simulink model "maquina_inducao_regime_permanente"  (R2015a)
settings: Solver=ode45  StartTime=0.0  StopTime=1.0  FixedStep=50e-6  MaxStep=50e-6  RelTol=1e-3
values from neighbouring files (symbols this model uses):
  FLrd_0 = FLr_dq_0    [MI_controle_W_I_T_inicio.m]    (also in MI_controle_W_I_inicio.m; MI_controle_W_I_startup_inicio.m; MI_controle_W_Inicio.m; MI_controle_W_T_I_startup_inicio.m)
  FLrq_0 = FluxLinkage_dq(4)    [MI_controle_W_I_T_inicio.m]    (also in MI_controle_W_I_inicio.m; MI_controle_W_I_startup_inicio.m; MI_controle_W_Inicio.m = 0; MI_controle_W_T_I_startup_inicio.m)
  FLsd_0 = FluxLinkage_dq(1)    [MI_controle_W_I_T_inicio.m]    (also in MI_controle_W_I_inicio.m; MI_controle_W_I_startup_inicio.m; MI_controle_W_Inicio.m; MI_controle_W_T_I_startup_inicio.m)
  FLsq_0 = FluxLinkage_dq(2)    [MI_controle_W_I_T_inicio.m]    (also in MI_controle_W_I_inicio.m; MI_controle_W_I_startup_inicio.m; MI_controle_W_Inicio.m; MI_controle_W_T_I_startup_inicio.m)
  J = 0.025    [MI_controle_W_I_T_inicio.m]    (also in MI_controle_W_I_inicio.m; MI_controle_W_I_startup_inicio.m; MI_controle_W_Inicio.m; MI_controle_W_T_I_startup_inicio.m)
  Lm = Xm/Wsyn    (= 0.368708951496)    [MI_controle_W_I_T_inicio.m]    (also in MI_controle_W_I_inicio.m; MI_controle_W_I_startup_inicio.m; MI_controle_W_Inicio.m; MI_controle_W_T_I_startup_inicio.m)
  Minv = inv(M)    [MI_controle_W_I_T_inicio.m]    (also in MI_controle_W_I_inicio.m; MI_controle_W_I_startup_inicio.m; MI_controle_W_Inicio.m; MI_controle_W_T_I_startup_inicio.m)
  p = 4    [MI_controle_W_I_T_inicio.m]    (also in MI_controle_W_I_inicio.m; MI_controle_W_I_startup_inicio.m; MI_controle_W_Inicio.m; MI_controle_W_T_I_startup_inicio.m)
  Rr = 1.34    [MI_controle_W_I_T_inicio.m]    (also in MI_controle_W_I_inicio.m; MI_controle_W_I_startup_inicio.m; MI_controle_W_Inicio.m; MI_controle_W_T_I_startup_inicio.m)
  Rs = 1.77    [MI_controle_W_I_T_inicio.m]    (also in MI_controle_W_I_inicio.m; MI_controle_W_I_startup_inicio.m; MI_controle_W_Inicio.m; MI_controle_W_T_I_startup_inicio.m)
  TL_0 = Tem_0    [MI_controle_W_I_T_inicio.m]    (also in MI_controle_W_I_inicio.m; MI_controle_W_I_startup_inicio.m = 0; MI_controle_W_Inicio.m; MI_controle_W_T_I_startup_inicio.m = 0)
  Va = VLLrms*sqrt(2/3)    [MI_controle_W_I_T_inicio.m]    (also in MI_controle_W_I_inicio.m; MI_controle_W_I_startup_inicio.m; MI_controle_W_Inicio.m; MI_controle_W_T_I_startup_inicio.m)
  Wmech_0 = (2/p)*(1-s)*Wsyn    (= 185.253435597)    [MI_controle_W_I_T_inicio.m]    (also in MI_controle_W_I_inicio.m; MI_controle_W_I_startup_inicio.m = 0; MI_controle_W_Inicio.m; MI_controle_W_T_I_startup_inicio.m = 0)
  Wsyn = 2*pi*f    (= 376.991118431)    [MI_controle_W_I_T_inicio.m]    (also in MI_controle_W_I_inicio.m; MI_controle_W_I_startup_inicio.m; MI_controle_W_Inicio.m; MI_controle_W_T_I_startup_inicio.m)
settings Model: Creator=range  LastModifiedBy=range

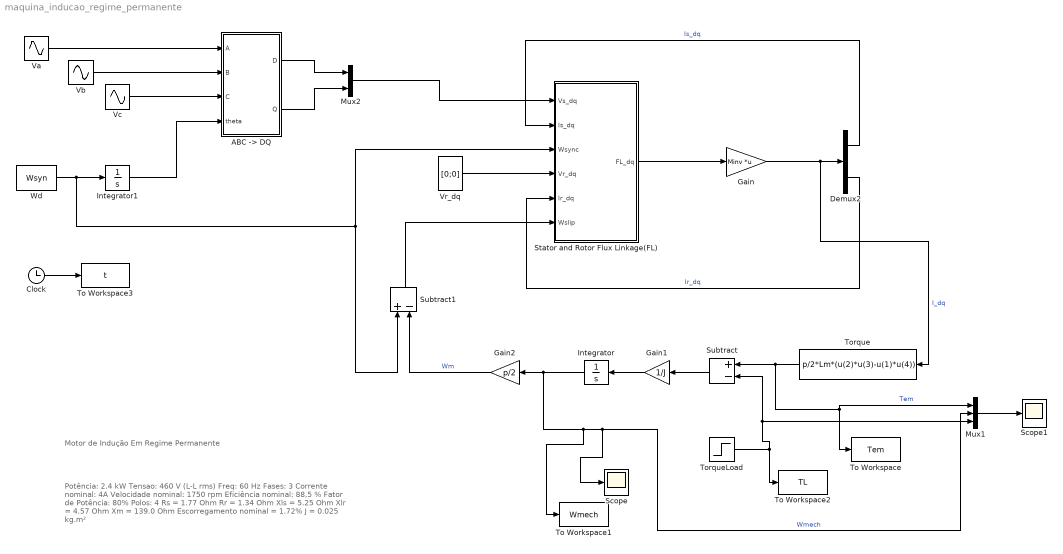
== system maquina_inducao_regime_permanente ==
  note: Potência: 2.4 kW
      | Tensao: 460 V (L-L rms)
      | Freq: 60 Hz
      | Fases: 3
      | Corrente nominal: 4A
      | Velocidade nominal: 1750 rpm
      | Eficiência nominal: 88,5 %
      | Fator de Potência: 80%
      | Polos: 4
      | Rs = 1.77 Ohm
      | Rr = 1.34 Ohm
      | Xls = 5.25 Ohm
      | Xlr = 4.57 Ohm
      | Xm = 139.0 Ohm
      | Escorregamento nominal = 1.72%
      | J = 0.025 kg.m²
  note: Motor de Indução Em Regime Permanente
  "ABC -> DQ" : MATLAB Function  TreatAsAtomicUnit=on
  Clock : Clock
  Demux2 : Demux  Outputs=2
  Gain : Gain  Gain=Minv  Multiplication=Matrix(K*u)
  Gain1 : Gain  Gain=1/J
  Gain2 : Gain  Gain=p/2
  Integrator : Integrator  InitialCondition=Wmech_0
  Integrator1 : Integrator
  Mux1 : Mux  Inputs=3
  Mux2 : Mux  Inputs=2
  Scope : Scope
      settings: YMin=375.5  YMax=378
  Scope1 : Scope
  "Stator and Rotor Flux Linkage(FL) " : Subsystem
  Subtract : Sum  Inputs=+-
  Subtract1 : Sum  Inputs=+-
  To Workspace : ToWorkspace  VariableName=Tem  SaveFormat=Timeseries  SampleTime=-1
  To Workspace1 : ToWorkspace  VariableName=Wmech  SaveFormat=Timeseries  SampleTime=-1
  To Workspace2 : ToWorkspace  VariableName=TL  SaveFormat=Timeseries  SampleTime=-1
  To Workspace3 : ToWorkspace  VariableName=t  SaveFormat=Timeseries  SampleTime=-1
  Torque : Fcn  Expr=p/2*Lm*(u(2)*u(3)-u(1)*u(4))
  TorqueLoad : Step  Time=0.1  Before=TL_0  After=TL_0/2  SampleTime=0
  Va : Sin  Amplitude=Va  Frequency=Wsyn  Phase=pi/2  SampleTime=0
  Vb : Sin  Amplitude=Va  Frequency=Wsyn  Phase=pi/2-2*pi/3  SampleTime=0
  Vc : Sin  Amplitude=Va  Frequency=Wsyn  Phase=pi/2-4*pi/3  SampleTime=0
  Vr_dq : Constant  Value=[0;0]  VectorParams1D=off
  Wd : Constant  Value=Wsyn
  wires:
  "Stator and Rotor Flux Linkage(FL) "/1(FL_dq) -> Gain/1
  Gain/1 -> Torque/1, Demux2/1  "I_dq"
  Vr_dq/1 -> "Stator and Rotor Flux Linkage(FL) "/4(Vr_dq)
  Demux2/1 -> "Stator and Rotor Flux Linkage(FL) "/2(Is_dq)  "Is_dq"
  Demux2/2 -> "Stator and Rotor Flux Linkage(FL) "/5(Ir_dq)  "Ir_dq"
  Torque/1 -> To Workspace/1, Mux1/1, Subtract/1  "Tem"
  TorqueLoad/1 -> Mux1/3, Subtract/2, To Workspace2/1
  Gain1/1 -> Integrator/1
  Subtract/1 -> Gain1/1
  Integrator/1 -> To Workspace1/1, Mux1/2, Scope/1, Gain2/1  "Wmech"
  Wd/1 -> Subtract1/1, "Stator and Rotor Flux Linkage(FL) "/3(Wsync), Integrator1/1
  Gain2/1 -> Subtract1/2  "Wm"
  Subtract1/1 -> "Stator and Rotor Flux Linkage(FL) "/6(Wslip)
  Clock/1 -> To Workspace3/1
  Mux1/1 -> Scope1/1
  Integrator1/1 -> "ABC -> DQ"/4(theta)
  Vc/1 -> "ABC -> DQ"/3(C)
  Vb/1 -> "ABC -> DQ"/2(B)
  Va/1 -> "ABC -> DQ"/1(A)
  "ABC -> DQ"/1(D) -> Mux2/1
  "ABC -> DQ"/2(Q) -> Mux2/2
  Mux2/1 -> "Stator and Rotor Flux Linkage(FL) "/1(Vs_dq)

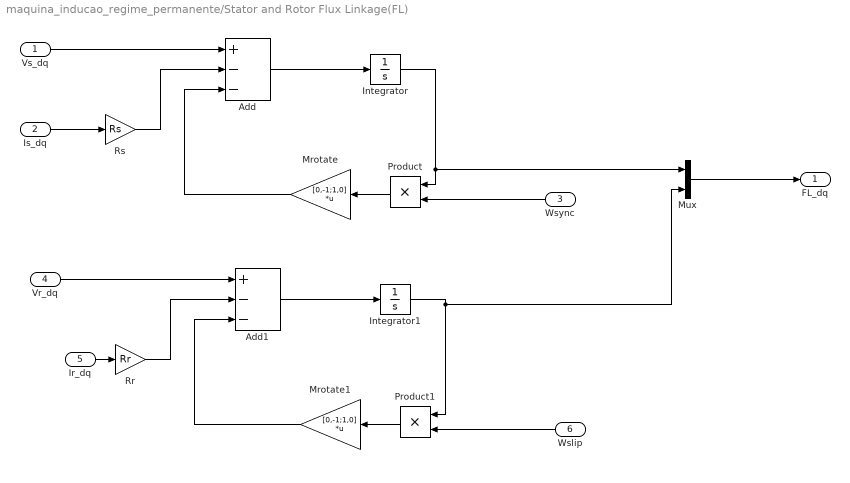
== system maquina_inducao_regime_permanente/Stator and Rotor Flux Linkage(FL)  ==
  Vs_dq : Inport
  Is_dq : Inport  Port=2
  Wsync : Inport  Port=3
  Vr_dq : Inport  Port=4
  Ir_dq : Inport  Port=5
  Wslip : Inport  Port=6
  Add : Sum  Inputs=+--
  Add1 : Sum  Inputs=+--
  Integrator : Integrator  InitialCondition=[FLsd_0;FLsq_0]
  Integrator1 : Integrator  InitialCondition=[FLrd_0;FLrq_0]
  Mrotate : Gain  Gain=[0,-1;1,0]  Multiplication=Matrix(K*u)
  Mrotate1 : Gain  Gain=[0,-1;1,0]  Multiplication=Matrix(K*u)
  Mux : Mux  Inputs=2
  Product : Product
  Product1 : Product
  Rr : Gain  Gain=Rr
  Rs : Gain  Gain=Rs
  FL_dq : Outport
  wires:
  Vs_dq/1 -> Add/1
  Product/1 -> Mrotate/1
  Rs/1 -> Add/2
  Add/1 -> Integrator/1
  Mrotate/1 -> Add/3
  Integrator/1 -> Mux/1, Product/1
  Wsync/1 -> Product/2
  Is_dq/1 -> Rs/1
  Vr_dq/1 -> Add1/1
  Product1/1 -> Mrotate1/1
  Rr/1 -> Add1/2
  Add1/1 -> Integrator1/1
  Mrotate1/1 -> Add1/3
  Integrator1/1 -> Mux/2, Product1/1
  Ir_dq/1 -> Rr/1
  Wslip/1 -> Product1/2
  Mux/1 -> FL_dq/1

== matlab function maquina_inducao_regime_permanente/ABC -> DQ ==
  data: A input; D output; B input; C input; theta input; Q output
function [D,Q] = ABCtoDQ(A,B,C,theta)
%Transformação de grandezas trifásicas para os eixos D e Q.

DQ = sqrt(2/3)*[cos(theta), cos(theta-2*pi/3), cos(theta-4*pi/3);...
               -sin(theta),-sin(theta-2*pi/3),-sin(theta-4*pi/3)]*[A;B;C];
D = DQ(1);
Q = DQ(2);
